simulink model "TestModel1"  (R2016b)
settings: Solver=ode1  StartTime=0.0  StopTime=10.0  FixedStep=0.01  RelTol=1e-3
libraries: simulink x2
settings Model: Creator=odj  LastModifiedBy=TSR2
settings DataIOCC: SaveFormat=StructureWithTime  ReturnWorkspaceOutputs=on
settings OptimizationCC: LifeSpan=inf
settings DebuggingCC: SolverPrmCheckMsg=warning  SFUnexpectedBacktrackingDiag=warning  SFNoUnconditionalDefaultTransitionDiag=warning  SFExecutionAtInitializationDiag=none
settings HardwareCC: ProdBitPerPointer=32  ProdBitPerSizeT=32  ProdBitPerPtrDiffT=32  ProdLargestAtomicFloat=None  ProdIntDivRoundTo=Undefined  ProdEndianess=Unspecified  ProdWordSize=32  ProdHWDeviceType=32-bit Generic  TargetBitPerPointer=64  TargetBitPerSizeT=64  TargetBitPerPtrDiffT=64  TargetLongLongMode=on  TargetIntDivRoundTo=Zero  TargetEndianess=LittleEndian  TargetWordSize=64  TargetHWDeviceType=MATLAB Host  ProdEqTarget=off
settings ModelReferenceCC: PropagateSignalLabelsOutOfModel=off
settings RTWCC: SystemTargetFile=rtwsfcnfmi.tlc  TemplateMakefile=rtwsfcnfmi_tmf  Description=S-Function Target with Functional Mockup Interface (FMI)
settings STFCustomTargetCC: ModelReferenceCompliant=off  CompOptLevelCompliant=on  GeneratePreprocessorConditionals=Disable all  MATLABClassNameForMDSCustomization=Simulink.SoftwareTarget.TargetSpecificTriggerConfigurationBase  SystemTargetFile=rtwsfcnfmi.tlc
settings ConfigComp: CovMetricSettings=dw  CovHtmlReporting=on  CovSaveCumulativeToWorkspaceVar=on  CovSaveSingleToWorkspaceVar=on  CovExternalEMLEnable=off  CovSFcnEnable=off

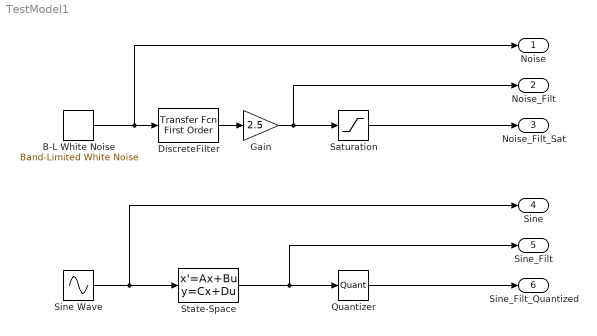
== system TestModel1 ==
  B-L White Noise : simulink/Sources/Band-Limited White Noise  Cov=[0.1]  Ts=0.05  seed=[23341]
  DiscreteFilter : simulink/Discrete/Transfer Fcn First Order  PoleZ=0.95  ICPrevOutput=0.0  DoSatur=off
  Gain : Gain  Gain=2.5
  Quantizer : Quantizer  QuantizationInterval=0.1  SampleTime=0.02
  Saturation : Saturate
  Sine Wave : Sin  Amplitude=2  SampleTime=0
  State-Space : StateSpace  A=[-4.2 -2.25;4 0]  B=[2 0]'  C=[0 1.125]  D=0  X0=0
  Noise : Outport
  Noise_Filt : Outport  Port=2
  Noise_Filt_Sat : Outport  Port=3
  Sine : Outport  Port=4
  Sine_Filt : Outport  Port=5
  Sine_Filt_Quantized : Outport  Port=6
  wires:
  B-L White Noise/1 -> DiscreteFilter/1, Noise/1
  DiscreteFilter/1 -> Gain/1
  Saturation/1 -> Noise_Filt_Sat/1
  Gain/1 -> Noise_Filt/1, Saturation/1
  Sine Wave/1 -> Sine/1, State-Space/1
  Quantizer/1 -> Sine_Filt_Quantized/1
  State-Space/1 -> Sine_Filt/1, Quantizer/1
